simulink model "ChiefMaster_TTC580"  (R2022b)
settings: Solver=FixedStepAuto  StartTime=0.0  StopTime=10  FixedStep=0.01  RelTol=1e-3
values from neighbouring files (symbols this model uses):
  BattBox1_No = single(1)    [Parameters.m]
  BattBox2_No = single(2)    [Parameters.m]
  BattBox3_No = single(3)    [Parameters.m]
  CurrentLB = single(-3)    [Parameters.m]
  CurrentReductionConstant_Lvl0 = single(0.03)    [Parameters.m]
  CurrentReductionConstant_Lvl1 = single(0.05)    [Parameters.m]
  CurrentReductionConstant_Lvl2 = single(0.07)    [Parameters.m]
  CurrentReductionConstant_Lvl3 = single(0.1)    [Parameters.m]
  CurrentUB = single(3)    [Parameters.m]
  DCHV_Minus_In_Delay_ms = single(500)    [Parameters.m]
  FL_sHVC_CellBalanceVoltage_mV = single(3500)    [Parameters.m]
  FL_sInrushCurrent_dividebyzero = single(0.00001)    [Parameters.m]
  FL_u8HMI_BuzzerTimer = uint8(3)    [Parameters.m]
  IP_boActValue = true    [Parameters.m]
  IP_boDeactValue = false    [Parameters.m]
  IP_boInitValue = false    [Parameters.m]
  IP_s_LB = 18000    [Parameters.m]
  IP_s_UB = 22000    [Parameters.m]
  IP_sBatt1_ChargeCurrentMax_Factor = single(0.1)    [Parameters.m]
  IP_sBatt1_ChargeCurrentMax_LB = single(0)    [Parameters.m]
  IP_sBatt1_ChargeCurrentMax_Offset = single(0)    [Parameters.m]
  IP_sBatt1_ChargeCurrentMax_UB = single(6553.5)    [Parameters.m]
  IP_sBatt1_Current_Factor = single(0.1)    [Parameters.m]
  IP_sBatt1_Current_LB = single(-3276.8)    [Parameters.m]
  IP_sBatt1_Current_Offset = single(0)    [Parameters.m]
  IP_sBatt1_Current_UB = single(3276.8)    [Parameters.m]
  IP_sBatt1_DisChargeCurrentMax_Factor = single(0.1)    [Parameters.m]
  IP_sBatt1_DisChargeCurrentMax_LB = single(0)    [Parameters.m]
  IP_sBatt1_DisChargeCurrentMax_Offset = single(0)    [Parameters.m]
  IP_sBatt1_DisChargeCurrentMax_UB = single(6553.5)    [Parameters.m]
  IP_sBatt1_InsulationResistance_Factor = single(5)    [Parameters.m]
  IP_sBatt1_InsulationResistance_LB = single(0)    [Parameters.m]
  IP_sBatt1_InsulationResistance_Offset = single(0)    [Parameters.m]
  IP_sBatt1_InsulationResistance_UB = single(0)    [Parameters.m]
  IP_sBatt1_LiBa_IntResist_mOhm = single(25)    [Parameters.m]
  IP_sBatt1_SOC_Factor = single(1)    [Parameters.m]
  IP_sBatt1_SOC_LB = single(0)    [Parameters.m]
  IP_sBatt1_SOC_Offset = single(0)    [Parameters.m]
  IP_sBatt1_SOC_UB = single(100)    [Parameters.m]
  IP_sBatt1_SOH_Factor = single(1)    [Parameters.m]
  IP_sBatt1_SOH_LB = single(0)    [Parameters.m]
  IP_sBatt1_SOH_Offset = single(0)    [Parameters.m]
  IP_sBatt1_SOH_UB = single(100)    [Parameters.m]
  IP_sBatt1_Ubatt_Factor = single(0.1)    [Parameters.m]
  IP_sBatt1_Ubatt_LB = single(0)    [Parameters.m]
  IP_sBatt1_Ubatt_Offset = single(0)    [Parameters.m]
  IP_sBatt1_Ubatt_UB = single(6553.5)    [Parameters.m]
  IP_sBatt1_UserRi_Factor = single(1)    [Parameters.m]
  IP_sBatt1_UserRi_LB = single(0)    [Parameters.m]
  IP_sBatt1_UserRi_Offset = single(0)    [Parameters.m]
  IP_sBatt1_UserRi_UB = single(255)    [Parameters.m]
  IP_sBatt1_VoltageAtSensor_Factor = single(0.02)    [Parameters.m]
  IP_sBatt1_VoltageAtSensor_LB = single(0)    [Parameters.m]
  IP_sBatt1_VoltageAtSensor_Offset = single(0)    [Parameters.m]
  IP_sBatt1_VoltageAtSensor_UB = single(1310.7)    [Parameters.m]
  IP_sBatt2_LiBa_IntResist_mOhm = single(25)    [Parameters.m]
  IP_sBatt3_LiBa_IntResist_mOhm = single(25)    [Parameters.m]
  IP_sEM_LB = 2000    [Parameters.m]
  IP_sEM_UB = 8000    [Parameters.m]
  IP_sFB_LB = 5000    [Parameters.m]
  IP_sFB_UB = 10000    [Parameters.m]
  IP_sHVIL_LB = 12000    [Parameters.m]
  IP_sHVIL_UB = 15000    [Parameters.m]
  IP_sLoad_Voltage_Factor = single(1)    [Parameters.m]
  IP_sLoad_Voltage_LB = single(0)    [Parameters.m]
  IP_sLoad_Voltage_Offset = single(0)    [Parameters.m]
  IP_sLoad_Voltage_UB = single(65535)    [Parameters.m]
  IP_u8HVIL_Delay_ms = uint8(100)    [Parameters.m]
  IP_u8HW_IN_delay_ms = uint8(100)    [Parameters.m]
  IT_sInsulationSafeValue_kOhm = single(650)    [Parameters.m]
  IT_u8IMD_DelayTime_s = uint8(20)    [Parameters.m]
  MainHV_Minus_In_Delay = single(5)    [Parameters.m]
  MainHV_StatusDelay = single(5)    [Parameters.m]
  NotAvailable_uint16 = single(65535)    [Parameters.m]
  NotAvailable_uint8 = uint8(255)    [Parameters.m]
  OP_boHVIL_Supply = boolean(1)    [Parameters.m]
  SafeCurrentToCloseHV_A = single(5)    [Parameters.m]
  SafeVoltageToCloseHV_V = single(0.5)    [Parameters.m]
  UnexpectedBattChargingFcn_Available = boolean(1)    [Parameters.m]
  Voltage_NA_UB = uint16(65535)    [Parameters.m]
  VoltageSensorAvailableBB1 = boolean(0)    [Parameters.m]
  VoltageSensorAvailableBB2 = boolean(0)    [Parameters.m]
  VoltageSensorAvailableBB3 = boolean(0)    [Parameters.m]
libraries: simulink x184, Library_DataProcessing_v1_1 x167, Library_DataProcessing_v1 x142, libCM x28
(part 13 of 19)

== system ChiefMaster_TTC580/ChiefMaster/Input Translation/Battery Signals/Subsystem9/Subsystem2 ==
  <IP_LB_BMS_IO_state_Input_DataBus> : Inport
  <IP_boBatt1_HV_relay_PLUS_Sense> : Inport  Port=2
  Bus Selector : BusSelector  OutputSignals=sData
  Compare To Constant : simulink/Logic and Bit Operations/Compare To Constant  relop===  const=128  OutDataTypeStr=boolean
  Compare To Constant1 : simulink/Logic and Bit Operations/Compare To Constant  relop===  const=160  OutDataTypeStr=boolean
  Compare To Constant2 : simulink/Logic and Bit Operations/Compare To Constant  relop===  const=224  OutDataTypeStr=boolean
  Constant : Constant  Value=0  OutDataTypeStr=boolean
  Multiport Switch : MultiPortSwitch  DataPortForDefault=Additional data port  DiagnosticForDefault=Warning  SaturateOnIntegerOverflow=off  InputSameDT=off
  OR : Logic  Operator=OR  Inputs=3  AllPortsSameDT=off  OutDataTypeStr=boolean
  IP_boBMS_HV_Plus_Sense_BB2 : Outport
  wires:
  OR/1 -> Multiport Switch/3
  <IP_LB_BMS_IO_state_Input_DataBus>/1 -> Bus Selector/1
  <IP_boBatt1_HV_relay_PLUS_Sense>/1 -> Multiport Switch/2
  Constant/1 -> Multiport Switch/5, Multiport Switch/4
  Bus Selector/1 -> Compare To Constant/1, Compare To Constant2/1, Compare To Constant1/1  "<sData>"
  [Select_Battery2] -> Multiport Switch/1
  Multiport Switch/1 -> IP_boBMS_HV_Plus_Sense_BB2/1  "IP_boBMS_HV_Plus_Sense_BB2"
  Compare To Constant1/1 -> OR/2
  Compare To Constant/1 -> OR/1
  Compare To Constant2/1 -> OR/3

== system ChiefMaster_TTC580/ChiefMaster/Input Translation/Battery Signals/Subsystem9/Subsystem3 ==
  <IP_boBatt2_HV_relay_MINUS_Sense> : Inport
  <IP_LB_BMS_IO_state_Input_DataBus> : Inport  Port=2
  Bus Selector : BusSelector  OutputSignals=sData
  Compare To Constant : simulink/Logic and Bit Operations/Compare To Constant  relop===  const=64  OutDataTypeStr=boolean
  Compare To Constant1 : simulink/Logic and Bit Operations/Compare To Constant  relop===  const=96  OutDataTypeStr=boolean
  Compare To Constant2 : simulink/Logic and Bit Operations/Compare To Constant  relop===  const=224  OutDataTypeStr=boolean
  Constant : Constant  Value=0  OutDataTypeStr=boolean
  Multiport Switch : MultiPortSwitch  DataPortForDefault=Additional data port  DiagnosticForDefault=Warning  SaturateOnIntegerOverflow=off  InputSameDT=off
  OR : Logic  Operator=OR  Inputs=3  AllPortsSameDT=off  OutDataTypeStr=boolean
  IP_boBMS_HV_Minus_Sense_BB2 : Outport
  wires:
  Multiport Switch/1 -> IP_boBMS_HV_Minus_Sense_BB2/1  "IP_boBMS_HV_Minus_Sense_BB2"
  [Select_Battery2] -> Multiport Switch/1
  Bus Selector/1 -> Compare To Constant/1, Compare To Constant2/1, Compare To Constant1/1  "<sData>"
  Constant/1 -> Multiport Switch/4, Multiport Switch/5
  <IP_boBatt2_HV_relay_MINUS_Sense>/1 -> Multiport Switch/2
  <IP_LB_BMS_IO_state_Input_DataBus>/1 -> Bus Selector/1
  OR/1 -> Multiport Switch/3
  Compare To Constant1/1 -> OR/2
  Compare To Constant/1 -> OR/1
  Compare To Constant2/1 -> OR/3

== system ChiefMaster_TTC580/ChiefMaster/Input Translation/Battery Signals/Subsystem9/Subsystem4 ==
  <IP_LB_BMS_IO_state_Input_DataBus> : Inport
  <IP_boBatt3_HV_relay_PLUS_Sense> : Inport  Port=2
  Bus Selector : BusSelector  OutputSignals=sData
  Compare To Constant : simulink/Logic and Bit Operations/Compare To Constant  relop===  const=128  OutDataTypeStr=boolean
  Compare To Constant1 : simulink/Logic and Bit Operations/Compare To Constant  relop===  const=160  OutDataTypeStr=boolean
  Compare To Constant2 : simulink/Logic and Bit Operations/Compare To Constant  relop===  const=224  OutDataTypeStr=boolean
  Constant : Constant  Value=0  OutDataTypeStr=boolean
  Multiport Switch : MultiPortSwitch  DataPortForDefault=Additional data port  DiagnosticForDefault=Warning  SaturateOnIntegerOverflow=off  InputSameDT=off
  OR : Logic  Operator=OR  Inputs=3  AllPortsSameDT=off  OutDataTypeStr=boolean
  IP_boBMS_HV_Plus_Sense_BB3 : Outport
  wires:
  Multiport Switch/1 -> IP_boBMS_HV_Plus_Sense_BB3/1  "IP_boBMS_HV_Plus_Sense_BB3"
  [Select_Battery3] -> Multiport Switch/1
  Bus Selector/1 -> Compare To Constant/1, Compare To Constant2/1, Compare To Constant1/1  "<sData>"
  Constant/1 -> Multiport Switch/4, Multiport Switch/5
  <IP_boBatt3_HV_relay_PLUS_Sense>/1 -> Multiport Switch/2
  <IP_LB_BMS_IO_state_Input_DataBus>/1 -> Bus Selector/1
  OR/1 -> Multiport Switch/3
  Compare To Constant1/1 -> OR/2
  Compare To Constant/1 -> OR/1
  Compare To Constant2/1 -> OR/3

== system ChiefMaster_TTC580/ChiefMaster/Input Translation/Battery Signals/Subsystem9/Subsystem5 ==
  <IP_boBatt3_HV_relay_MINUS_Sense> : Inport
  <IP_LB_BMS_IO_state_Input_DataBus> : Inport  Port=2
  Bus Selector : BusSelector  OutputSignals=sData
  Compare To Constant : simulink/Logic and Bit Operations/Compare To Constant  relop===  const=64  OutDataTypeStr=boolean
  Compare To Constant1 : simulink/Logic and Bit Operations/Compare To Constant  relop===  const=96  OutDataTypeStr=boolean
  Compare To Constant2 : simulink/Logic and Bit Operations/Compare To Constant  relop===  const=224  OutDataTypeStr=boolean
  Constant : Constant  Value=0  OutDataTypeStr=boolean
  Multiport Switch : MultiPortSwitch  DataPortForDefault=Additional data port  DiagnosticForDefault=Warning  SaturateOnIntegerOverflow=off  InputSameDT=off
  OR : Logic  Operator=OR  Inputs=3  AllPortsSameDT=off  OutDataTypeStr=boolean
  IP_boBMS_HV_Minus_Sense_BB3 : Outport
  wires:
  OR/1 -> Multiport Switch/3
  <IP_LB_BMS_IO_state_Input_DataBus>/1 -> Bus Selector/1
  <IP_boBatt3_HV_relay_MINUS_Sense>/1 -> Multiport Switch/2
  Constant/1 -> Multiport Switch/5, Multiport Switch/4
  Bus Selector/1 -> Compare To Constant/1, Compare To Constant2/1, Compare To Constant1/1  "<sData>"
  [Select_Battery3] -> Multiport Switch/1
  Multiport Switch/1 -> IP_boBMS_HV_Minus_Sense_BB3/1  "IP_boBMS_HV_Minus_Sense_BB3"
  Compare To Constant1/1 -> OR/2
  Compare To Constant/1 -> OR/1
  Compare To Constant2/1 -> OR/3

== system ChiefMaster_TTC580/ChiefMaster/Input Translation/Battery Signals/Subsystem9/Subsystem8 ==
  <IP_boBatt1_HV_relay_MINUS_Sense> : Inport
  <IP_LB_BMS_IO_state_Input_DataBus> : Inport  Port=2
  Bus Selector : BusSelector  OutputSignals=sData
  Compare To Constant : simulink/Logic and Bit Operations/Compare To Constant  relop===  const=64  OutDataTypeStr=boolean
  Compare To Constant1 : simulink/Logic and Bit Operations/Compare To Constant  relop===  const=96  OutDataTypeStr=boolean
  Compare To Constant2 : simulink/Logic and Bit Operations/Compare To Constant  relop===  const=224  OutDataTypeStr=boolean
  Constant : Constant  Value=0  OutDataTypeStr=boolean
  Multiport Switch : MultiPortSwitch  DataPortForDefault=Additional data port  DiagnosticForDefault=Warning  SaturateOnIntegerOverflow=off  InputSameDT=off
  OR : Logic  Operator=OR  Inputs=3  AllPortsSameDT=off  OutDataTypeStr=boolean
  IP_boBMS_HV_Minus_Sense_BB1 : Outport
  wires:
  Multiport Switch/1 -> IP_boBMS_HV_Minus_Sense_BB1/1  "IP_boBMS_HV_Minus_Sense_BB1"
  [Select_Battery1] -> Multiport Switch/1
  Bus Selector/1 -> Compare To Constant/1, Compare To Constant2/1, Compare To Constant1/1  "<sData>"
  Constant/1 -> Multiport Switch/4, Multiport Switch/5
  <IP_boBatt1_HV_relay_MINUS_Sense>/1 -> Multiport Switch/2
  <IP_LB_BMS_IO_state_Input_DataBus>/1 -> Bus Selector/1
  OR/1 -> Multiport Switch/3
  Compare To Constant/1 -> OR/1
  Compare To Constant1/1 -> OR/2
  Compare To Constant2/1 -> OR/3

== system ChiefMaster_TTC580/ChiefMaster/Output Processing/CM_OBD/CM_BDU_Msg5_6/Subsystem1 ==
  Calculated_InrushCurr_BB2 : Inport
  Constant : Constant  Value=0  OutDataTypeStr=single
  Constant1 : Constant  Value=0.1  OutDataTypeStr=single
  Lib_2bytes_Split1 : Library_DataProcessing_v1/Lib_2bytes_Split  SystemSampleTime=-1  VariantActivationTime=update diagram  Latency=0  AutoFrameSizeCalculation=off
  Lib_OutProcessing1 : Library_DataProcessing_v1/Lib_OutProcessing  SystemSampleTime=-1  VariantActivationTime=update diagram  Latency=0  AutoFrameSizeCalculation=off
  u8byte_LSB : Outport
  u8byte_MSB : Outport  Port=2
  wires:
  Constant1/1 -> Lib_OutProcessing1/3
  Constant/1 -> Lib_OutProcessing1/2
  Lib_2bytes_Split1/1 -> u8byte_LSB/1
  Lib_2bytes_Split1/2 -> u8byte_MSB/1
  Calculated_InrushCurr_BB2/1 -> Lib_OutProcessing1/1
  Lib_OutProcessing1/1 -> Lib_2bytes_Split1/1

== system ChiefMaster_TTC580/ChiefMaster/Output Processing/CM_OBD/CM_BDU_Msg5_6/Subsystem4 ==
  Calculated_VtgDiff_BB1 : Inport
  Constant : Constant  Value=0  OutDataTypeStr=single
  Constant1 : Constant  Value=0.1  OutDataTypeStr=single
  Lib_2bytes_Split1 : Library_DataProcessing_v1/Lib_2bytes_Split  SystemSampleTime=-1  VariantActivationTime=update diagram  Latency=0  AutoFrameSizeCalculation=off
  Lib_OutProcessing1 : Library_DataProcessing_v1/Lib_OutProcessing  SystemSampleTime=-1  VariantActivationTime=update diagram  Latency=0  AutoFrameSizeCalculation=off
  u8byte_LSB : Outport
  u8byte_MSB : Outport  Port=2
  wires:
  Lib_OutProcessing1/1 -> Lib_2bytes_Split1/1
  Calculated_VtgDiff_BB1/1 -> Lib_OutProcessing1/1
  Lib_2bytes_Split1/2 -> u8byte_MSB/1
  Lib_2bytes_Split1/1 -> u8byte_LSB/1
  Constant/1 -> Lib_OutProcessing1/2
  Constant1/1 -> Lib_OutProcessing1/3

== system ChiefMaster_TTC580/ChiefMaster/Output Processing/CM_OBD/CM_BDU_Msg5_6/Subsystem5 ==
  Calculated_VtgDiff_BB2 : Inport
  Constant : Constant  Value=0  OutDataTypeStr=single
  Constant1 : Constant  Value=0.1  OutDataTypeStr=single
  Lib_2bytes_Split1 : Library_DataProcessing_v1/Lib_2bytes_Split  SystemSampleTime=-1  VariantActivationTime=update diagram  Latency=0  AutoFrameSizeCalculation=off
  Lib_OutProcessing1 : Library_DataProcessing_v1/Lib_OutProcessing  SystemSampleTime=-1  VariantActivationTime=update diagram  Latency=0  AutoFrameSizeCalculation=off
  u8byte_LSB : Outport
  u8byte_MSB : Outport  Port=2
  wires:
  Constant1/1 -> Lib_OutProcessing1/3
  Constant/1 -> Lib_OutProcessing1/2
  Lib_2bytes_Split1/1 -> u8byte_LSB/1
  Lib_2bytes_Split1/2 -> u8byte_MSB/1
  Calculated_VtgDiff_BB2/1 -> Lib_OutProcessing1/1
  Lib_OutProcessing1/1 -> Lib_2bytes_Split1/1

== system ChiefMaster_TTC580/ChiefMaster/Output Processing/CM_OBD/CM_BDU_Msg5_6/Subsystem6 ==
  Calculated_VtgDiff_BB3 : Inport
  Constant : Constant  Value=0  OutDataTypeStr=single
  Constant1 : Constant  Value=0.1  OutDataTypeStr=single
  Lib_2bytes_Split1 : Library_DataProcessing_v1/Lib_2bytes_Split  SystemSampleTime=-1  VariantActivationTime=update diagram  Latency=0  AutoFrameSizeCalculation=off
  Lib_OutProcessing1 : Library_DataProcessing_v1/Lib_OutProcessing  SystemSampleTime=-1  VariantActivationTime=update diagram  Latency=0  AutoFrameSizeCalculation=off
  u8byte_LSB : Outport
  u8byte_MSB : Outport  Port=2
  wires:
  Lib_OutProcessing1/1 -> Lib_2bytes_Split1/1
  Calculated_VtgDiff_BB3/1 -> Lib_OutProcessing1/1
  Lib_2bytes_Split1/2 -> u8byte_MSB/1
  Lib_2bytes_Split1/1 -> u8byte_LSB/1
  Constant/1 -> Lib_OutProcessing1/2
  Constant1/1 -> Lib_OutProcessing1/3

== system ChiefMaster_TTC580/ChiefMaster/Output Processing/CM_OBD/CM_BDU_Msg5_6/Subsystem8 ==
  Calculated_InrushCurr_BB2 : Inport
  Constant : Constant  Value=0  OutDataTypeStr=single
  Constant1 : Constant  Value=0.1  OutDataTypeStr=single
  Lib_2bytes_Split1 : Library_DataProcessing_v1/Lib_2bytes_Split  SystemSampleTime=-1  VariantActivationTime=update diagram  Latency=0  AutoFrameSizeCalculation=off
  Lib_OutProcessing1 : Library_DataProcessing_v1/Lib_OutProcessing  SystemSampleTime=-1  VariantActivationTime=update diagram  Latency=0  AutoFrameSizeCalculation=off
  u8byte_LSB : Outport
  u8byte_MSB : Outport  Port=2
  wires:
  Lib_OutProcessing1/1 -> Lib_2bytes_Split1/1
  Calculated_InrushCurr_BB2/1 -> Lib_OutProcessing1/1
  Lib_2bytes_Split1/2 -> u8byte_MSB/1
  Lib_2bytes_Split1/1 -> u8byte_LSB/1
  Constant/1 -> Lib_OutProcessing1/2
  Constant1/1 -> Lib_OutProcessing1/3

== system ChiefMaster_TTC580/ChiefMaster/Output Processing/CM_OBD/CM_BDU_Msg5_6/Subsystem9 ==
  Calculated_InrushCurr_BB3 : Inport
  Constant : Constant  Value=0  OutDataTypeStr=single
  Constant1 : Constant  Value=0.1  OutDataTypeStr=single
  Lib_2bytes_Split1 : Library_DataProcessing_v1/Lib_2bytes_Split  SystemSampleTime=-1  VariantActivationTime=update diagram  Latency=0  AutoFrameSizeCalculation=off
  Lib_OutProcessing1 : Library_DataProcessing_v1/Lib_OutProcessing  SystemSampleTime=-1  VariantActivationTime=update diagram  Latency=0  AutoFrameSizeCalculation=off
  u8byte_LSB : Outport
  u8byte_MSB : Outport  Port=2
  wires:
  Constant1/1 -> Lib_OutProcessing1/3
  Constant/1 -> Lib_OutProcessing1/2
  Lib_2bytes_Split1/1 -> u8byte_LSB/1
  Lib_2bytes_Split1/2 -> u8byte_MSB/1
  Calculated_InrushCurr_BB3/1 -> Lib_OutProcessing1/1
  Lib_OutProcessing1/1 -> Lib_2bytes_Split1/1

== system ChiefMaster_TTC580/ChiefMaster/Output Processing/CM_OBD/CM_IP_Msg1/LoadVoltage ==
  LoadVoltage : Inport  OutDataTypeStr=single
  Constant2 : Constant  Value=0.1  OutDataTypeStr=single
  Constant4 : Constant  Value=0  OutDataTypeStr=single
  Lib_2bytes_Split1 : Library_DataProcessing_v1/Lib_2bytes_Split  SystemSampleTime=-1  VariantActivationTime=update diagram  Latency=0  AutoFrameSizeCalculation=off
  Lib_OutProcessing1 : Library_DataProcessing_v1/Lib_OutProcessing  SystemSampleTime=-1  VariantActivationTime=update diagram  Latency=0  AutoFrameSizeCalculation=off
  u8byte_LSB : Outport
  u8byte_MSB : Outport  Port=2
  wires:
  Lib_OutProcessing1/1 -> Lib_2bytes_Split1/1
  Constant2/1 -> Lib_OutProcessing1/3
  Constant4/1 -> Lib_OutProcessing1/2
  LoadVoltage/1 -> Lib_OutProcessing1/1
  Lib_2bytes_Split1/2 -> u8byte_MSB/1
  Lib_2bytes_Split1/1 -> u8byte_LSB/1

== system ChiefMaster_TTC580/ChiefMaster/Output Processing/CM_OBD/CM_SystemStatus1_Msg3/Subsystem ==
  IP_DataBus : Inport
  Constant2 : Constant  Value=FL_sHVC_CellBalanceVoltage_mV
  Subsystem12 : Subsystem
  fcn_HVCellBalanceCheck : Subsystem  ReferencedSubsystem=fcn_HVCellBalanceCheck
      settings: RTWFcnNameOpts=Use subsystem name  RTWFileNameOpts=Use subsystem name
  FL_boHVC_AllCellBalanced : Outport
  wires:
  Constant2/1 -> fcn_HVCellBalanceCheck/1, Subsystem12/1(FL_sHVC_CellBalanceVoltage_mV)
  fcn_HVCellBalanceCheck/1 -> FL_boHVC_AllCellBalanced/1
  Subsystem12/3(Batt3_UCellMin) -> fcn_HVCellBalanceCheck/4
  Subsystem12/1(Batt1_UCellMin) -> fcn_HVCellBalanceCheck/2
  Subsystem12/2(Batt2_UCellMin) -> fcn_HVCellBalanceCheck/3
  IP_DataBus/1 -> Subsystem12/2(IP_DataBus)

== system ChiefMaster_TTC580/ChiefMaster/Output Processing/CM_OBD/CM_SystemStatus2_Msg4/Subsystem ==
  System_Current : Inport
  Constant : Constant  Value=0  OutDataTypeStr=single
  Constant1 : Constant  Value=0.1  OutDataTypeStr=single
  Lib_2bytes_Split1 : Library_DataProcessing_v1/Lib_2bytes_Split  SystemSampleTime=-1  VariantActivationTime=update diagram  Latency=0  AutoFrameSizeCalculation=off
  Lib_OutProcessing1 : Library_DataProcessing_v1/Lib_OutProcessing  SystemSampleTime=-1  VariantActivationTime=update diagram  Latency=0  AutoFrameSizeCalculation=off
  u8byte_LSB : Outport
  u8byte_MSB : Outport  Port=2
  wires:
  Lib_OutProcessing1/1 -> Lib_2bytes_Split1/1
  System_Current/1 -> Lib_OutProcessing1/1
  Lib_2bytes_Split1/2 -> u8byte_MSB/1
  Lib_2bytes_Split1/1 -> u8byte_LSB/1
  Constant/1 -> Lib_OutProcessing1/2
  Constant1/1 -> Lib_OutProcessing1/3

== system ChiefMaster_TTC580/ChiefMaster/Output Processing/CM_OBD/CM_SystemStatus2_Msg4/Subsystem1 ==
  System_Voltage : Inport
  Constant : Constant  Value=0  OutDataTypeStr=single
  Constant1 : Constant  OutDataTypeStr=single
  Lib_2bytes_Split1 : Library_DataProcessing_v1/Lib_2bytes_Split  SystemSampleTime=-1  VariantActivationTime=update diagram  Latency=0  AutoFrameSizeCalculation=off
  Lib_OutProcessing1 : Library_DataProcessing_v1/Lib_OutProcessing  SystemSampleTime=-1  VariantActivationTime=update diagram  Latency=0  AutoFrameSizeCalculation=off
  u8byte_LSB : Outport
  u8byte_MSB : Outport  Port=2
  wires:
  Constant1/1 -> Lib_OutProcessing1/3
  Constant/1 -> Lib_OutProcessing1/2
  Lib_2bytes_Split1/1 -> u8byte_LSB/1
  Lib_2bytes_Split1/2 -> u8byte_MSB/1
  System_Voltage/1 -> Lib_OutProcessing1/1
  Lib_OutProcessing1/1 -> Lib_2bytes_Split1/1

== system ChiefMaster_TTC580/ChiefMaster/Output Processing/CM_OBD/CM_SystemStatus2_Msg4/Subsystem2 ==
  MaxChargeCurrent : Inport
  Constant : Constant  Value=0  OutDataTypeStr=single
  Constant1 : Constant  OutDataTypeStr=single
  Lib_2bytes_Split1 : Library_DataProcessing_v1/Lib_2bytes_Split  SystemSampleTime=-1  VariantActivationTime=update diagram  Latency=0  AutoFrameSizeCalculation=off
  Lib_OutProcessing1 : Library_DataProcessing_v1/Lib_OutProcessing  SystemSampleTime=-1  VariantActivationTime=update diagram  Latency=0  AutoFrameSizeCalculation=off
  u8byte_LSB : Outport
  u8byte_MSB : Outport  Port=2
  wires:
  Lib_OutProcessing1/1 -> Lib_2bytes_Split1/1
  MaxChargeCurrent/1 -> Lib_OutProcessing1/1
  Lib_2bytes_Split1/2 -> u8byte_MSB/1
  Lib_2bytes_Split1/1 -> u8byte_LSB/1
  Constant/1 -> Lib_OutProcessing1/2
  Constant1/1 -> Lib_OutProcessing1/3

== system ChiefMaster_TTC580/ChiefMaster/Output Processing/CM_OBD/CM_SystemStatus2_Msg4/Subsystem3 ==
  MaxDisChargeCurrent : Inport
  Constant : Constant  Value=0  OutDataTypeStr=single
  Constant1 : Constant  OutDataTypeStr=single
  Lib_2bytes_Split1 : Library_DataProcessing_v1/Lib_2bytes_Split  SystemSampleTime=-1  VariantActivationTime=update diagram  Latency=0  AutoFrameSizeCalculation=off
  Lib_OutProcessing1 : Library_DataProcessing_v1/Lib_OutProcessing  SystemSampleTime=-1  VariantActivationTime=update diagram  Latency=0  AutoFrameSizeCalculation=off
  u8byte_LSB : Outport
  u8byte_MSB : Outport  Port=2
  wires:
  Constant1/1 -> Lib_OutProcessing1/3
  Constant/1 -> Lib_OutProcessing1/2
  Lib_2bytes_Split1/1 -> u8byte_LSB/1
  Lib_2bytes_Split1/2 -> u8byte_MSB/1
  MaxDisChargeCurrent/1 -> Lib_OutProcessing1/1
  Lib_OutProcessing1/1 -> Lib_2bytes_Split1/1

== system ChiefMaster_TTC580/ChiefMaster/Input Processing/Actia/Batt Box 1/Subsystem1/Subsystem3 ==
  byte1 : Inport
  byte2 : Inport  Port=2
  C_Batt1_ADS_3_560_Timeout : Inport  Port=3
  Bus Creator : BusCreator  Inputs=3
  Constant : Constant  Value=IP_sBatt1_Ubatt_Factor  OutDataTypeStr=single
  Constant1 : Constant  Value=IP_sBatt1_Ubatt_Offset  OutDataTypeStr=single
  Constant2 : Constant  Value=IP_sBatt1_Ubatt_LB  OutDataTypeStr=single
  Constant3 : Constant  Value=IP_sBatt1_Ubatt_UB  OutDataTypeStr=single
  Lib_2byte_ArthConcat : Library_DataProcessing_v1/Lib_2byte_ArthConcat  SystemSampleTime=-1  VariantActivationTime=update diagram  Latency=0  AutoFrameSizeCalculation=off
  Lib_InputProcessing+SafeValueSelector_Data : Library_DataProcessing_v1/Lib_InputProcessing+SafeValueSelector_Data  SystemSampleTime=-1  VariantActivationTime=update diagram  Latency=0  AutoFrameSizeCalculation=off
  SafeValue_Error : Constant  Priority=1005  Value=0  OutDataTypeStr=single
  "SafeValue_NA " : Constant  Priority=1006  Value=0  OutDataTypeStr=single
  IP_sBatt1_Ubatt_Databus : Outport
  wires:
  Lib_2byte_ArthConcat/1 -> Lib_InputProcessing+SafeValueSelector_Data/1
  C_Batt1_ADS_3_560_Timeout/1 -> Lib_InputProcessing+SafeValueSelector_Data/2
  "SafeValue_NA "/1 -> Lib_InputProcessing+SafeValueSelector_Data/8
  Lib_InputProcessing+SafeValueSelector_Data/1 -> Bus Creator/1
  SafeValue_Error/1 -> Lib_InputProcessing+SafeValueSelector_Data/7
  Lib_InputProcessing+SafeValueSelector_Data/2 -> Bus Creator/2
  Lib_InputProcessing+SafeValueSelector_Data/3 -> Bus Creator/3
  Constant3/1 -> Lib_InputProcessing+SafeValueSelector_Data/6
  Constant2/1 -> Lib_InputProcessing+SafeValueSelector_Data/5
  Constant/1 -> Lib_InputProcessing+SafeValueSelector_Data/3
  Constant1/1 -> Lib_InputProcessing+SafeValueSelector_Data/4
  byte2/1 -> Lib_2byte_ArthConcat/2
  byte1/1 -> Lib_2byte_ArthConcat/1
  Bus Creator/1 -> IP_sBatt1_Ubatt_Databus/1  "IP_sBatt1_Ubatt_Databus"

== system ChiefMaster_TTC580/ChiefMaster/Input Processing/Actia/Batt Box 1/Subsystem2/Subsystem ==
  byte1 : Inport
  Timeout : EnablePort
  Bus Creator : BusCreator  Inputs=7
  Data Type Conversion{2..8} (7 alike) : DataTypeConversion  OutDataTypeStr=boolean  SaturateOnIntegerOverflow=off  RndMeth=Floor
  Extract Bits : simulink/Logic and Bit Operations/Extract Bits  bitsToExtract=Range of bits  numBits=8  bitIdxRange=[0]  outScalingMode=Treat bit field as an integer
  Extract Bits1 : simulink/Logic and Bit Operations/Extract Bits  bitsToExtract=Range of bits  numBits=8  bitIdxRange=[1]  outScalingMode=Treat bit field as an integer
  Extract Bits2 : simulink/Logic and Bit Operations/Extract Bits  bitsToExtract=Range of bits  numBits=8  bitIdxRange=[2]  outScalingMode=Treat bit field as an integer
  Extract Bits3 : simulink/Logic and Bit Operations/Extract Bits  bitsToExtract=Range of bits  numBits=8  bitIdxRange=[3]  outScalingMode=Treat bit field as an integer
  Extract Bits4 : simulink/Logic and Bit Operations/Extract Bits  bitsToExtract=Range of bits  numBits=8  bitIdxRange=[4]  outScalingMode=Treat bit field as an integer
  Extract Bits5 : simulink/Logic and Bit Operations/Extract Bits  bitsToExtract=Range of bits  numBits=8  bitIdxRange=[5]  outScalingMode=Treat bit field as an integer
  Extract Bits6 : simulink/Logic and Bit Operations/Extract Bits  bitsToExtract=Range of bits  numBits=8  bitIdxRange=[6]  outScalingMode=Treat bit field as an integer
  Batt1_MyStatus1_Databus : Outport  OutputWhenDisabled=reset  InitialOutput=[0]
  wires:
  Extract Bits5/1 -> Data Type Conversion7/1
  byte1/1 -> Extract Bits4/1, Extract Bits5/1, Extract Bits6/1, Extract Bits/1, Extract Bits1/1, Extract Bits2/1, Extract Bits3/1
  Extract Bits3/1 -> Data Type Conversion5/1
  Extract Bits6/1 -> Data Type Conversion8/1
  Extract Bits/1 -> Data Type Conversion2/1
  Extract Bits1/1 -> Data Type Conversion3/1
  Extract Bits4/1 -> Data Type Conversion6/1
  Extract Bits2/1 -> Data Type Conversion4/1
  Data Type Conversion2/1 -> Bus Creator/1  "IP_boBatt1_HV_REL_ON"
  Data Type Conversion3/1 -> Bus Creator/2  "IP_boBatt1_HV_REL_OFF"
  Data Type Conversion4/1 -> Bus Creator/3  "IP_boBatt1_Insulation_Relay_ON"
  Data Type Conversion5/1 -> Bus Creator/4  "IP_boBatt1_SDERR_activ"
  Data Type Conversion6/1 -> Bus Creator/5  "IP_boBatt1_ERROR_activ"
  Data Type Conversion7/1 -> Bus Creator/6  "IP_boBatt1_WARNING_activ"
  Data Type Conversion8/1 -> Bus Creator/7  "IP_boBatt1_Insulation_ready_and_OK"
  Bus Creator/1 -> Batt1_MyStatus1_Databus/1  "Batt1_MyStatus1_Databus"

== system ChiefMaster_TTC580/ChiefMaster/Input Processing/Actia/Batt Box 1/Subsystem2/Subsystem2 ==
  byte2 : Inport
  byte3 : Inport  Port=2
  C_Actia_Batt1_MyStatus_Timeout : Inport  Port=3
  Bus Creator : BusCreator  Inputs=3
  Constant : Constant  Value=IP_sBatt1_DisChargeCurrentMax_Factor  OutDataTypeStr=single
  Constant1 : Constant  Value=IP_sBatt1_DisChargeCurrentMax_Offset  OutDataTypeStr=single
  Constant2 : Constant  Value=IP_sBatt1_DisChargeCurrentMax_LB  OutDataTypeStr=single
  Constant3 : Constant  Value=IP_sBatt1_DisChargeCurrentMax_UB  OutDataTypeStr=single
  Lib_2byte_ArthConcat : Library_DataProcessing_v1/Lib_2byte_ArthConcat  SystemSampleTime=-1  VariantActivationTime=update diagram  Latency=0  AutoFrameSizeCalculation=off
  Lib_InputProcessing+SafeValueSelector_Data : Library_DataProcessing_v1/Lib_InputProcessing+SafeValueSelector_Data  SystemSampleTime=-1  VariantActivationTime=update diagram  Latency=0  AutoFrameSizeCalculation=off
  SafeValue_Error : Constant  Priority=1005  Value=0  OutDataTypeStr=single
  "SafeValue_NA " : Constant  Priority=1006  Value=0  OutDataTypeStr=single
  IP_sBatt1_DisChargeCurrentMax_A_Databus : Outport
  wires:
  Bus Creator/1 -> IP_sBatt1_DisChargeCurrentMax_A_Databus/1  "IP_sBatt1_DisChargeCurrentMax_A_Databus"
  byte2/1 -> Lib_2byte_ArthConcat/1
  byte3/1 -> Lib_2byte_ArthConcat/2
  Constant1/1 -> Lib_InputProcessing+SafeValueSelector_Data/4
  Constant/1 -> Lib_InputProcessing+SafeValueSelector_Data/3
  Constant2/1 -> Lib_InputProcessing+SafeValueSelector_Data/5
  Constant3/1 -> Lib_InputProcessing+SafeValueSelector_Data/6
  Lib_InputProcessing+SafeValueSelector_Data/3 -> Bus Creator/3
  Lib_InputProcessing+SafeValueSelector_Data/2 -> Bus Creator/2
  SafeValue_Error/1 -> Lib_InputProcessing+SafeValueSelector_Data/7
  Lib_InputProcessing+SafeValueSelector_Data/1 -> Bus Creator/1
  "SafeValue_NA "/1 -> Lib_InputProcessing+SafeValueSelector_Data/8
  C_Actia_Batt1_MyStatus_Timeout/1 -> Lib_InputProcessing+SafeValueSelector_Data/2
  Lib_2byte_ArthConcat/1 -> Lib_InputProcessing+SafeValueSelector_Data/1

== system ChiefMaster_TTC580/ChiefMaster/Input Processing/Actia/Batt Box 1/Subsystem2/Subsystem3 ==
  byte2 : Inport
  byte3 : Inport  Port=2
  C_Actia_Batt1_MyStatus_Timeout : Inport  Port=3
  Bus Creator : BusCreator  Inputs=3
  Constant : Constant  Value=IP_sBatt1_VoltageAtSensor_Factor  OutDataTypeStr=single
  Constant1 : Constant  Value=IP_sBatt1_VoltageAtSensor_Offset  OutDataTypeStr=single
  Constant2 : Constant  Value=IP_sBatt1_VoltageAtSensor_LB  OutDataTypeStr=single
  Constant3 : Constant  Value=IP_sBatt1_VoltageAtSensor_UB  OutDataTypeStr=single
  Lib_2byte_ArthConcat : Library_DataProcessing_v1/Lib_2byte_ArthConcat  SystemSampleTime=-1  VariantActivationTime=update diagram  Latency=0  AutoFrameSizeCalculation=off
  Lib_InputProcessing+SafeValueSelector_Data : Library_DataProcessing_v1/Lib_InputProcessing+SafeValueSelector_Data  SystemSampleTime=-1  VariantActivationTime=update diagram  Latency=0  AutoFrameSizeCalculation=off
  SafeValue_Error : Constant  Priority=1005  Value=0  OutDataTypeStr=single
  "SafeValue_NA " : Constant  Priority=1006  Value=0  OutDataTypeStr=single
  IP_sBatt1_VoltageAtSensor_V_Databus : Outport
  wires:
  Lib_2byte_ArthConcat/1 -> Lib_InputProcessing+SafeValueSelector_Data/1
  C_Actia_Batt1_MyStatus_Timeout/1 -> Lib_InputProcessing+SafeValueSelector_Data/2
  "SafeValue_NA "/1 -> Lib_InputProcessing+SafeValueSelector_Data/8
  Lib_InputProcessing+SafeValueSelector_Data/1 -> Bus Creator/1
  SafeValue_Error/1 -> Lib_InputProcessing+SafeValueSelector_Data/7
  Lib_InputProcessing+SafeValueSelector_Data/2 -> Bus Creator/2
  Lib_InputProcessing+SafeValueSelector_Data/3 -> Bus Creator/3
  Constant3/1 -> Lib_InputProcessing+SafeValueSelector_Data/6
  Constant2/1 -> Lib_InputProcessing+SafeValueSelector_Data/5
  Constant/1 -> Lib_InputProcessing+SafeValueSelector_Data/3
  Constant1/1 -> Lib_InputProcessing+SafeValueSelector_Data/4
  byte3/1 -> Lib_2byte_ArthConcat/2
  byte2/1 -> Lib_2byte_ArthConcat/1
  Bus Creator/1 -> IP_sBatt1_VoltageAtSensor_V_Databus/1  "IP_sBatt1_VoltageAtSensor_V_Databus"

== system ChiefMaster_TTC580/ChiefMaster/Input Processing/Actia/Batt Box 1/Subsystem2/Subsystem4 ==
  byte2 : Inport
  byte3 : Inport  Port=2
  C_Actia_Batt1_MyStatus_Timeout : Inport  Port=3
  Bus Creator : BusCreator  Inputs=3
  Constant : Constant  Value=IP_sBatt1_ChargeCurrentMax_Factor  OutDataTypeStr=single
  Constant1 : Constant  Value=IP_sBatt1_ChargeCurrentMax_Offset  OutDataTypeStr=single
  Constant2 : Constant  Value=IP_sBatt1_ChargeCurrentMax_LB  OutDataTypeStr=single
  Constant3 : Constant  Value=IP_sBatt1_ChargeCurrentMax_UB  OutDataTypeStr=single
  Lib_2byte_ArthConcat : Library_DataProcessing_v1/Lib_2byte_ArthConcat  SystemSampleTime=-1  VariantActivationTime=update diagram  Latency=0  AutoFrameSizeCalculation=off
  Lib_InputProcessing+SafeValueSelector_Data : Library_DataProcessing_v1/Lib_InputProcessing+SafeValueSelector_Data  SystemSampleTime=-1  VariantActivationTime=update diagram  Latency=0  AutoFrameSizeCalculation=off
  SafeValue_Error : Constant  Priority=1005  Value=0  OutDataTypeStr=single
  "SafeValue_NA " : Constant  Priority=1006  Value=0  OutDataTypeStr=single
  IP_sBatt1_ChargeCurrentMax_A_Databus : Outport
  wires:
  Lib_2byte_ArthConcat/1 -> Lib_InputProcessing+SafeValueSelector_Data/1
  C_Actia_Batt1_MyStatus_Timeout/1 -> Lib_InputProcessing+SafeValueSelector_Data/2
  "SafeValue_NA "/1 -> Lib_InputProcessing+SafeValueSelector_Data/8
  Lib_InputProcessing+SafeValueSelector_Data/1 -> Bus Creator/1
  SafeValue_Error/1 -> Lib_InputProcessing+SafeValueSelector_Data/7
  Lib_InputProcessing+SafeValueSelector_Data/2 -> Bus Creator/2
  Lib_InputProcessing+SafeValueSelector_Data/3 -> Bus Creator/3
  Constant3/1 -> Lib_InputProcessing+SafeValueSelector_Data/6
  Constant2/1 -> Lib_InputProcessing+SafeValueSelector_Data/5
  Constant/1 -> Lib_InputProcessing+SafeValueSelector_Data/3
  Constant1/1 -> Lib_InputProcessing+SafeValueSelector_Data/4
  byte3/1 -> Lib_2byte_ArthConcat/2
  byte2/1 -> Lib_2byte_ArthConcat/1
  Bus Creator/1 -> IP_sBatt1_ChargeCurrentMax_A_Databus/1  "IP_sBatt1_ChargeCurrentMax_A_Databus"

== system ChiefMaster_TTC580/ChiefMaster/Input Processing/Actia/Batt Box 1/Subsystem3/Subsystem1 ==
  byte4 : Inport
  byte5 : Inport  Port=2
  C_BMS500_Timeout : Inport  Port=3
  Bus Creator : BusCreator  Inputs=3
  Constant4 : Constant  OutDataTypeStr=single
  Constant{5..6,8..9} (4 alike) : Constant  Value=0  OutDataTypeStr=single
  Constant7 : Constant  Value=4500  OutDataTypeStr=single
  Lib_2byte_ArthConcat : Library_DataProcessing_v1_1/Lib_2byte_ArthConcat  SystemSampleTime=-1  VariantActivationTime=update diagram  Latency=0  AutoFrameSizeCalculation=off
  Lib_InputProcessing+SafeValueSelector_Data : Library_DataProcessing_v1_1/Lib_InputProcessing+SafeValueSelector_Data  SystemSampleTime=-1  VariantActivationTime=update diagram  Latency=0  AutoFrameSizeCalculation=off
  IP_sActia_Batt1_MinCellVolt_mV_DataBus : Outport
  wires:
  byte5/1 -> Lib_2byte_ArthConcat/2
  byte4/1 -> Lib_2byte_ArthConcat/1
  Bus Creator/1 -> IP_sActia_Batt1_MinCellVolt_mV_DataBus/1  "IP_sActia_Batt1_MinCellVolt_mV_DataBus"
  Lib_InputProcessing+SafeValueSelector_Data/3 -> Bus Creator/3
  Constant9/1 -> Lib_InputProcessing+SafeValueSelector_Data/8
  Lib_InputProcessing+SafeValueSelector_Data/2 -> Bus Creator/2
  Constant7/1 -> Lib_InputProcessing+SafeValueSelector_Data/6
  Constant6/1 -> Lib_InputProcessing+SafeValueSelector_Data/5
  Constant8/1 -> Lib_InputProcessing+SafeValueSelector_Data/7
  Lib_2byte_ArthConcat/1 -> Lib_InputProcessing+SafeValueSelector_Data/1
  Constant5/1 -> Lib_InputProcessing+SafeValueSelector_Data/4
  Constant4/1 -> Lib_InputProcessing+SafeValueSelector_Data/3
  C_BMS500_Timeout/1 -> Lib_InputProcessing+SafeValueSelector_Data/2
  Lib_InputProcessing+SafeValueSelector_Data/1 -> Bus Creator/1

== system ChiefMaster_TTC580/ChiefMaster/Input Processing/Actia/Batt Box 1/Subsystem3/Subsystem2 ==
  byte6 : Inport
  byte7 : Inport  Port=2
  C_BMS500_Timeout : Inport  Port=3
  Bus Creator : BusCreator  Inputs=3
  Constant4 : Constant  OutDataTypeStr=single
  Constant{5..6,8..9} (4 alike) : Constant  Value=0  OutDataTypeStr=single
  Constant7 : Constant  Value=4500  OutDataTypeStr=single
  Lib_2byte_ArthConcat : Library_DataProcessing_v1_1/Lib_2byte_ArthConcat  SystemSampleTime=-1  VariantActivationTime=update diagram  Latency=0  AutoFrameSizeCalculation=off
  Lib_InputProcessing+SafeValueSelector_Data : Library_DataProcessing_v1_1/Lib_InputProcessing+SafeValueSelector_Data  SystemSampleTime=-1  VariantActivationTime=update diagram  Latency=0  AutoFrameSizeCalculation=off
  IP_sActia_Batt1_MaxCellVolt_mV_DataBus : Outport
  wires:
  Bus Creator/1 -> IP_sActia_Batt1_MaxCellVolt_mV_DataBus/1  "IP_sActia_Batt1_MaxCellVolt_mV_DataBus"
  byte6/1 -> Lib_2byte_ArthConcat/1
  byte7/1 -> Lib_2byte_ArthConcat/2
  C_BMS500_Timeout/1 -> Lib_InputProcessing+SafeValueSelector_Data/2
  Constant4/1 -> Lib_InputProcessing+SafeValueSelector_Data/3
  Constant5/1 -> Lib_InputProcessing+SafeValueSelector_Data/4
  Constant8/1 -> Lib_InputProcessing+SafeValueSelector_Data/7
  Constant6/1 -> Lib_InputProcessing+SafeValueSelector_Data/5
  Lib_InputProcessing+SafeValueSelector_Data/2 -> Bus Creator/2
  Constant9/1 -> Lib_InputProcessing+SafeValueSelector_Data/8
  Lib_InputProcessing+SafeValueSelector_Data/3 -> Bus Creator/3
  Lib_2byte_ArthConcat/1 -> Lib_InputProcessing+SafeValueSelector_Data/1
  Lib_InputProcessing+SafeValueSelector_Data/1 -> Bus Creator/1
  Constant7/1 -> Lib_InputProcessing+SafeValueSelector_Data/6

== system ChiefMaster_TTC580/ChiefMaster/Input Processing/Actia/Batt Box 1/Subsystem4/Subsystem ==
  byte7 : Inport
  Timeout : EnablePort
  Data Type Conversion{2..5} (4 alike) : DataTypeConversion  OutDataTypeStr=boolean  SaturateOnIntegerOverflow=off  RndMeth=Floor
  Extract Bits : simulink/Logic and Bit Operations/Extract Bits  bitsToExtract=Range of bits  numBits=8  bitIdxRange=[0]  outScalingMode=Treat bit field as an integer
  Extract Bits1 : simulink/Logic and Bit Operations/Extract Bits  bitsToExtract=Range of bits  numBits=8  bitIdxRange=[1]  outScalingMode=Treat bit field as an integer
  Extract Bits2 : simulink/Logic and Bit Operations/Extract Bits  bitsToExtract=Range of bits  numBits=8  bitIdxRange=[2]  outScalingMode=Treat bit field as an integer
  Extract Bits3 : simulink/Logic and Bit Operations/Extract Bits  bitsToExtract=Range of bits  numBits=8  bitIdxRange=[4]  outScalingMode=Treat bit field as an integer
  IP_boBatt1_HV_relay_PLUS_Sense : Outport  OutputWhenDisabled=reset  InitialOutput=[0]
  IP_boBatt1_HV_PRECHARGE_active : Outport  Port=2  OutputWhenDisabled=reset  InitialOutput=[0]
  IP_boBatt1_HV_relay_MINUS_Sense : Outport  Port=3  OutputWhenDisabled=reset  InitialOutput=[0]
  IP_boBatt1_IMD_active : Outport  Port=4  OutputWhenDisabled=reset  InitialOutput=[0]
  wires:
  Data Type Conversion5/1 -> IP_boBatt1_IMD_active/1  "IP_boBatt1_IMD_active"
  Data Type Conversion4/1 -> IP_boBatt1_HV_relay_MINUS_Sense/1  "IP_boBatt1_HV_relay_MINUS_Sense"
  Data Type Conversion3/1 -> IP_boBatt1_HV_PRECHARGE_active/1  "IP_boBatt1_HV_PRECHARGE_active"
  Data Type Conversion2/1 -> IP_boBatt1_HV_relay_PLUS_Sense/1  "IP_boBatt1_HV_relay_PLUS_Sense"
  Extract Bits2/1 -> Data Type Conversion4/1
  Extract Bits1/1 -> Data Type Conversion3/1
  Extract Bits/1 -> Data Type Conversion2/1
  Extract Bits3/1 -> Data Type Conversion5/1
  byte7/1 -> Extract Bits3/1, Extract Bits2/1, Extract Bits1/1, Extract Bits/1

== system ChiefMaster_TTC580/ChiefMaster/Input Processing/Actia/Batt Box 1/Subsystem4/Subsystem1 ==
  byte8 : Inport
  Timeout : EnablePort
  Data Type Conversion6 : DataTypeConversion  OutDataTypeStr=boolean  SaturateOnIntegerOverflow=off  RndMeth=Floor
  Data Type Conversion7 : DataTypeConversion  OutDataTypeStr=boolean  SaturateOnIntegerOverflow=off  RndMeth=Floor
  Data Type Conversion8 : DataTypeConversion  OutDataTypeStr=boolean  SaturateOnIntegerOverflow=off  RndMeth=Floor
  Extract Bits : simulink/Logic and Bit Operations/Extract Bits  bitsToExtract=Range of bits  numBits=8  bitIdxRange=[0]  outScalingMode=Treat bit field as an integer
  Extract Bits1 : simulink/Logic and Bit Operations/Extract Bits  bitsToExtract=Range of bits  numBits=8  bitIdxRange=[1]  outScalingMode=Treat bit field as an integer
  Extract Bits2 : simulink/Logic and Bit Operations/Extract Bits  bitsToExtract=Range of bits  numBits=8  bitIdxRange=[2]  outScalingMode=Treat bit field as an integer
  IP_boBatt1_Drive_Mode_active : Outport  OutputWhenDisabled=reset  InitialOutput=[0]
  IP_boBatt1_PlugIn_Mode_active : Outport  Port=2  OutputWhenDisabled=reset  InitialOutput=[0]
  IP_boBatt1_Charging_finished : Outport  Port=3  OutputWhenDisabled=reset  InitialOutput=[0]
  wires:
  byte8/1 -> Extract Bits2/1, Extract Bits/1, Extract Bits1/1
  Extract Bits/1 -> Data Type Conversion6/1
  Extract Bits1/1 -> Data Type Conversion7/1
  Extract Bits2/1 -> Data Type Conversion8/1
  Data Type Conversion7/1 -> IP_boBatt1_PlugIn_Mode_active/1  "IP_boBatt1_PlugIn_Mode_active"
  Data Type Conversion6/1 -> IP_boBatt1_Drive_Mode_active/1  "IP_boBatt1_Drive_Mode_active"
  Data Type Conversion8/1 -> IP_boBatt1_Charging_finished/1  "IP_boBatt1_Charging_finished"

== system ChiefMaster_TTC580/ChiefMaster/Input Processing/Actia/Batt Box 1/Subsystem4/Subsystem2 ==
  byte2 : Inport
  Timeout : EnablePort
  Data Type Conversion2 : DataTypeConversion  OutDataTypeStr=boolean  SaturateOnIntegerOverflow=off  RndMeth=Floor
  Extract Bits : simulink/Logic and Bit Operations/Extract Bits  bitsToExtract=Range of bits  numBits=8  bitIdxRange=[0]  outScalingMode=Treat bit field as an integer
  IP_boBatt1_SDErr_SecuritySwitch : Outport  OutputWhenDisabled=reset  InitialOutput=[0]
  wires:
  byte2/1 -> Extract Bits/1
  Extract Bits/1 -> Data Type Conversion2/1
  Data Type Conversion2/1 -> IP_boBatt1_SDErr_SecuritySwitch/1  "IP_boBatt1_SDErr_SecuritySwitch"

== system ChiefMaster_TTC580/ChiefMaster/Input Processing/Actia/Batt Box 1/Subsystem5/Subsystem ==
  byte6 : Inport
  C_Batt1_ADS_8_600_Timeout : Inport  Port=2
  Bus Creator : BusCreator  Inputs=3
  Constant : Constant  Priority=983  Value=IP_sBatt1_InsulationResistance_Factor  OutDataTypeStr=single
  Constant1 : Constant  Priority=984  Value=IP_sBatt1_InsulationResistance_Offset  OutDataTypeStr=single
  Constant2 : Constant  Priority=985  Value=IP_sBatt1_InsulationResistance_LB  OutDataTypeStr=single
  Constant3 : Constant  Priority=986  Value=IP_sBatt1_InsulationResistance_UB  OutDataTypeStr=single
  Lib_InputProcessing+SafeValueSelector_Data : Library_DataProcessing_v1/Lib_InputProcessing+SafeValueSelector_Data  SystemSampleTime=-1  VariantActivationTime=update diagram  Latency=0  AutoFrameSizeCalculation=off
  SafeValue_Error : Constant  Priority=987  Value=0  OutDataTypeStr=single
  "SafeValue_NA " : Constant  Priority=988  Value=0  OutDataTypeStr=single
  IP_sBatt1_InsulationResistance_kOhms_DataBus : Outport
  wires:
  C_Batt1_ADS_8_600_Timeout/1 -> Lib_InputProcessing+SafeValueSelector_Data/2
  "SafeValue_NA "/1 -> Lib_InputProcessing+SafeValueSelector_Data/8
  Lib_InputProcessing+SafeValueSelector_Data/1 -> Bus Creator/1
  SafeValue_Error/1 -> Lib_InputProcessing+SafeValueSelector_Data/7
  Lib_InputProcessing+SafeValueSelector_Data/2 -> Bus Creator/2
  Lib_InputProcessing+SafeValueSelector_Data/3 -> Bus Creator/3
  byte6/1 -> Lib_InputProcessing+SafeValueSelector_Data/1
  Constant3/1 -> Lib_InputProcessing+SafeValueSelector_Data/6
  Constant2/1 -> Lib_InputProcessing+SafeValueSelector_Data/5
  Constant1/1 -> Lib_InputProcessing+SafeValueSelector_Data/4
  Constant/1 -> Lib_InputProcessing+SafeValueSelector_Data/3
  Bus Creator/1 -> IP_sBatt1_InsulationResistance_kOhms_DataBus/1  "IP_sBatt1_InsulationResistance_kOhms_DataBus"

== system ChiefMaster_TTC580/ChiefMaster/Input Processing/Actia/Batt Box 1/Subsystem5/Subsystem1 ==
  byte7 : Inport
  C_Batt1_ADS_8_600_Timeout : Inport  Port=2
  Bus Creator : BusCreator  Inputs=3
  Constant : Constant  Priority=983  Value=IP_sBatt1_SOC_Factor  OutDataTypeStr=single
  Constant1 : Constant  Priority=984  Value=IP_sBatt1_SOC_Offset  OutDataTypeStr=single
  Constant2 : Constant  Priority=985  Value=IP_sBatt1_SOC_LB  OutDataTypeStr=single
  Constant3 : Constant  Priority=986  Value=IP_sBatt1_SOC_UB  OutDataTypeStr=single
  Lib_InputProcessing+SafeValueSelector_Data : Library_DataProcessing_v1/Lib_InputProcessing+SafeValueSelector_Data  SystemSampleTime=-1  VariantActivationTime=update diagram  Latency=0  AutoFrameSizeCalculation=off
  SafeValue_Error : Constant  Priority=987  Value=0  OutDataTypeStr=single
  "SafeValue_NA " : Constant  Priority=988  Value=0  OutDataTypeStr=single
  IP_sBatt1_SOC_percent_DataBus : Outport
  wires:
  Bus Creator/1 -> IP_sBatt1_SOC_percent_DataBus/1  "IP_sBatt1_SOC_percent_DataBus"
  Constant/1 -> Lib_InputProcessing+SafeValueSelector_Data/3
  Constant1/1 -> Lib_InputProcessing+SafeValueSelector_Data/4
  Constant2/1 -> Lib_InputProcessing+SafeValueSelector_Data/5
  Constant3/1 -> Lib_InputProcessing+SafeValueSelector_Data/6
  byte7/1 -> Lib_InputProcessing+SafeValueSelector_Data/1
  Lib_InputProcessing+SafeValueSelector_Data/3 -> Bus Creator/3
  Lib_InputProcessing+SafeValueSelector_Data/2 -> Bus Creator/2
  SafeValue_Error/1 -> Lib_InputProcessing+SafeValueSelector_Data/7
  Lib_InputProcessing+SafeValueSelector_Data/1 -> Bus Creator/1
  "SafeValue_NA "/1 -> Lib_InputProcessing+SafeValueSelector_Data/8
  C_Batt1_ADS_8_600_Timeout/1 -> Lib_InputProcessing+SafeValueSelector_Data/2

== system ChiefMaster_TTC580/ChiefMaster/Input Processing/Actia/Batt Box 1/Subsystem5/Subsystem2 ==
  byte4 : Inport
  byte5 : Inport  Port=2
  C_Batt1_ADS_8_600_Timeout : Inport  Port=3
  Bus Creator : BusCreator  Inputs=3
  Constant : Constant  Value=IP_sBatt1_Current_Factor  OutDataTypeStr=single
  Constant1 : Constant  Value=IP_sBatt1_Current_Offset  OutDataTypeStr=single
  Constant2 : Constant  Value=IP_sBatt1_Current_LB  OutDataTypeStr=single
  Constant3 : Constant  Value=IP_sBatt1_Current_UB  OutDataTypeStr=single
  Lib_2byte_i16ArthConcat : Library_DataProcessing_v1/Lib_2byte_i16ArthConcat  SystemSampleTime=-1  VariantActivationTime=update diagram  Latency=0  AutoFrameSizeCalculation=off
  Lib_InputProcessing+SafeValueSelector_Data : Library_DataProcessing_v1/Lib_InputProcessing+SafeValueSelector_Data  SystemSampleTime=-1  VariantActivationTime=update diagram  Latency=0  AutoFrameSizeCalculation=off
  SafeValue_Error : Constant  Priority=1011  Value=0  OutDataTypeStr=single
  "SafeValue_NA " : Constant  Priority=1012  Value=0  OutDataTypeStr=single
  IP_sBatt1_Current_A_DataBus : Outport
  wires:
  Lib_2byte_i16ArthConcat/1 -> Lib_InputProcessing+SafeValueSelector_Data/1
  C_Batt1_ADS_8_600_Timeout/1 -> Lib_InputProcessing+SafeValueSelector_Data/2
  "SafeValue_NA "/1 -> Lib_InputProcessing+SafeValueSelector_Data/8
  Lib_InputProcessing+SafeValueSelector_Data/1 -> Bus Creator/1
  SafeValue_Error/1 -> Lib_InputProcessing+SafeValueSelector_Data/7
  Lib_InputProcessing+SafeValueSelector_Data/2 -> Bus Creator/2
  Lib_InputProcessing+SafeValueSelector_Data/3 -> Bus Creator/3
  Constant3/1 -> Lib_InputProcessing+SafeValueSelector_Data/6
  Constant2/1 -> Lib_InputProcessing+SafeValueSelector_Data/5
  Constant/1 -> Lib_InputProcessing+SafeValueSelector_Data/3
  Constant1/1 -> Lib_InputProcessing+SafeValueSelector_Data/4
  byte5/1 -> Lib_2byte_i16ArthConcat/2
  byte4/1 -> Lib_2byte_i16ArthConcat/1
  Bus Creator/1 -> IP_sBatt1_Current_A_DataBus/1  "IP_sBatt1_Current_A_DataBus"

== system ChiefMaster_TTC580/ChiefMaster/Input Processing/Actia/Batt Box 1/Subsystem5/Subsystem3 ==
  byte8 : Inport
  C_Batt1_ADS_8_600_Timeout : Inport  Port=2
  Bus Creator : BusCreator  Inputs=3
  Constant : Constant  Priority=983  Value=IP_sBatt1_SOH_Factor  OutDataTypeStr=single
  Constant1 : Constant  Priority=984  Value=IP_sBatt1_SOH_Offset  OutDataTypeStr=single
  Constant2 : Constant  Priority=985  Value=IP_sBatt1_SOH_LB  OutDataTypeStr=single
  Constant3 : Constant  Priority=986  Value=IP_sBatt1_SOH_UB  OutDataTypeStr=single
  Lib_InputProcessing+SafeValueSelector_Data : Library_DataProcessing_v1/Lib_InputProcessing+SafeValueSelector_Data  SystemSampleTime=-1  VariantActivationTime=update diagram  Latency=0  AutoFrameSizeCalculation=off
  SafeValue_Error : Constant  Priority=987  Value=0  OutDataTypeStr=single
  "SafeValue_NA " : Constant  Priority=988  Value=0  OutDataTypeStr=single
  IP_sBatt1_SOH_percent_DataBus : Outport
  wires:
  C_Batt1_ADS_8_600_Timeout/1 -> Lib_InputProcessing+SafeValueSelector_Data/2
  "SafeValue_NA "/1 -> Lib_InputProcessing+SafeValueSelector_Data/8
  Lib_InputProcessing+SafeValueSelector_Data/1 -> Bus Creator/1
  SafeValue_Error/1 -> Lib_InputProcessing+SafeValueSelector_Data/7
  Lib_InputProcessing+SafeValueSelector_Data/2 -> Bus Creator/2
  Lib_InputProcessing+SafeValueSelector_Data/3 -> Bus Creator/3
  byte8/1 -> Lib_InputProcessing+SafeValueSelector_Data/1
  Constant3/1 -> Lib_InputProcessing+SafeValueSelector_Data/6
  Constant2/1 -> Lib_InputProcessing+SafeValueSelector_Data/5
  Constant1/1 -> Lib_InputProcessing+SafeValueSelector_Data/4
  Constant/1 -> Lib_InputProcessing+SafeValueSelector_Data/3
  Bus Creator/1 -> IP_sBatt1_SOH_percent_DataBus/1  "IP_sBatt1_SOH_percent_DataBus"
